simulink model "Model_1"  (R2020b)
settings: Solver=VariableStepAuto  StartTime=0.0  StopTime=10.0  RelTol=1e-3
values from neighbouring files (symbols this model uses):
  C = 0.000001    (= 1e-06)    [S1.m]
  R = 10    [S1.m]
settings Model: Creator=Diwakar Reddy  LastModifiedBy=Diwakar Reddy

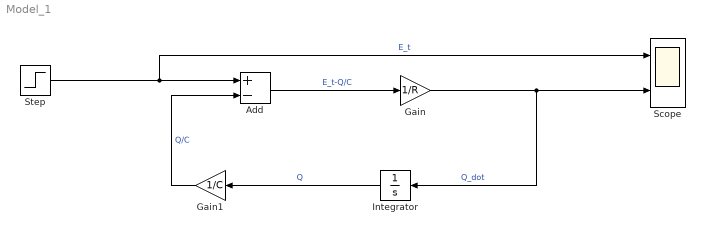
== system Model_1 ==
  Add : Sum  Inputs=+-
  Gain : Gain  Gain=1/R
  Gain1 : Gain  Gain=1/C
  Integrator : Integrator
  Scope : Scope  NumInputPorts=2
  Step : Step  SampleTime=0
  wires:
  Gain/1 -> Integrator/1, Scope/2  "Q_dot"
  Step/1 -> Scope/1, Add/1  "E_t"
  Add/1 -> Gain/1  "E_t-Q/C"
  Integrator/1 -> Gain1/1  "Q"
  Gain1/1 -> Add/2  "Q/C"
